simulink model "Gleichstrommaschine"  (R2016a)
settings: Solver=ode15s  SolverMode=SingleTasking  StartTime=0  StopTime=40  FixedStep=T_tast  MaxStep=0.8  RelTol=1e-9
PreLoadFcn:
  | ,try, xsg_acmc_mdl_preloadfcn(bdroot, 'LoadModel'); catch, disp(lasterr); end,
PostLoadFcn:
  | , if any(exist('dsrtsu_mdlpostloadfcn', 'file') == [2, 3, 6]), try dsrtsu_mdlpostloadfcn('Execute', bdroot); catch fprintf('Error in PostLoadFcn (dsrtsu_mdlpostloadfcn) for model "%s":\n %s\n', bdroot, lasterr); end, end,
  | ,try, xsg_acmc_mdl_postloadfcn(bdroot, 'UpdateModel', 170100); catch, disp(lasterr); end,
undefined symbols (not defined in the file): J, km, Lq, Rq, Ud
PreSaveFcn:
  | , if any(exist('dsmpb_private', 'file') == [2, 3, 6]), try, dsmpb_private('dsmpb_mdlclblib', 'PreSave', bdroot); catch, disp(lasterr); end, end,
CloseFcn:
  | , if any(exist('dsmpb_private', 'file') == [2, 3, 6]), try, dsmpb_private('dsmpb_mdlclblib', 'Close', bdroot); catch, disp(lasterr); end, end,
Description:
  | Standard RTI1202 template.
  | Supported Matlab version:  R2017a.
settings Model: Tag=RTI1202  DSRTSU_INTERNAL_RTI_VER=500  DSRTSU_INTERNAL_RTI_TYPE=rti1202  DSRTSU_INTERNAL_RTIFPGA=90  DSMPB_DATASERVER_ModelPortLibVersion1=8  DSMPB_DATASERVER_DataServerVersion1=6  DSMPB_DATASERVER_DataServerStreamVersion1=3  Creator=adminbochmann  LastModifiedBy=schreiner
settings OptimizationCC: BlockReduction=off  OptimizeBlockIOStorage=off  BufferReuse=off  GlobalBufferReuse=off  ExpressionFolding=off  LocalBlockOutputs=off
settings DebuggingCC: MultiTaskRateTransMsg=warning  SFUnexpectedBacktrackingDiag=error  SFNoUnconditionalDefaultTransitionDiag=error
settings HardwareCC: ProdBitPerPointer=32  ProdLargestAtomicInteger=Integer  ProdEndianess=BigEndian  ProdWordSize=32  ProdHWDeviceType=Custom Processor->Custom  TargetIntDivRoundTo=Zero  TargetEndianess=BigEndian  TargetHWDeviceType=Custom Processor->Custom
settings RTWCC: SystemTargetFile=rti1202.tlc  MakeCommand=make_rti  TemplateMakefile=rti1202.tmf  Description=dSPACE DS1202 Hardware Platform
settings STFCustomTargetCC: ParMdlRefBuildCompliant=on  GRTInterface=off  SystemTargetFile=rti1202.tlc
settings GRTTargetCC: CompOptLevelCompliant=off  ConcurrentExecutionCompliant=off  GeneratePreprocessorConditionals=Use local settings  CombineOutputUpdateFcns=off  MatFileLogging=off  CPPClassGenCompliant=off  UseToolchainInfoCompliant=off
settings ConfigComp: CovMetricSettings=dswe  CovHtmlReporting=off  CovSaveCumulativeToWorkspaceVar=off  CovSaveSingleToWorkspaceVar=off  CovExternalEMLEnable=on

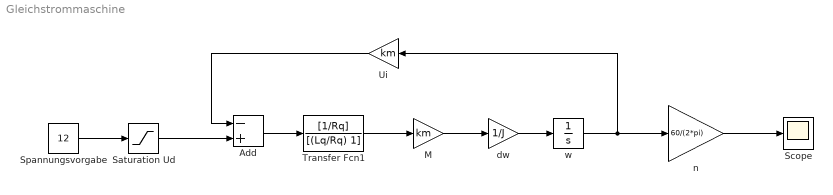
== system Gleichstrommaschine ==
  Add : Sum  Inputs=-+
  M : Gain  Gain=km
  Saturation Ud : Saturate  UpperLimit=Ud  LowerLimit=-Ud
  Scope : Scope
  Spannungsvorgabe : Constant  Value=12
  Transfer Fcn1 : TransferFcn  Numerator=[1/Rq]  Denominator=[(Lq/Rq) 1]
  Ui : Gain  Gain=km
  "dw " : Gain  Gain=1/J
  "n " : Gain  Gain=60/(2*pi)
  w : Integrator
  wires:
  "dw "/1 -> w/1
  M/1 -> "dw "/1
  Transfer Fcn1/1 -> M/1
  Saturation Ud/1 -> Add/2
  w/1 -> Ui/1, "n "/1
  Spannungsvorgabe/1 -> Saturation Ud/1
  "n "/1 -> Scope/1
  Add/1 -> Transfer Fcn1/1
  Ui/1 -> Add/1
